simulink model "DirectSequenceSpreadSpectrumCommunicationSystemSimulation"  (R2023a)
settings: Solver=VariableStepAuto  StartTime=0.0  StopTime=10  RelTol=1e-3
InitFcn:
  | fs=1e4;
  | Ts=1/fs;
  | Tb=0.1;
  | Tc=0.0125;
  | frame_size=1000;
libraries: commdigbbndpm3 x4, dspsrcs4 x4, commrandsrc3 x2, commfilt2 x2, commchan3 x1, dspstat3 x1
settings Model: Creator=STUDENT  LastModifiedBy=LENOVO
settings SolverCC: AlgebraicLoopSolver=TrustRegion
settings DebuggingCC: UnconnectedInputMsg=warning  UnconnectedOutputMsg=warning  UnconnectedLineMsg=warning
settings ModelReferenceCC: EnableRefExpFcnMdlSchedulingChecks=on
settings SFSimCC: CustomCodeUndefinedFunction=UseInterfaceOnly

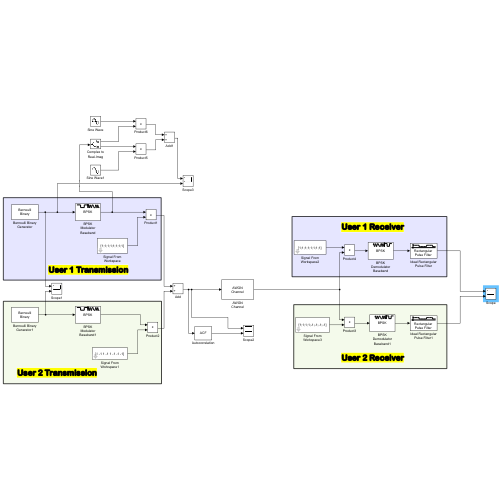
[thumbnail: Simulink's stored preview of the top-level diagram]
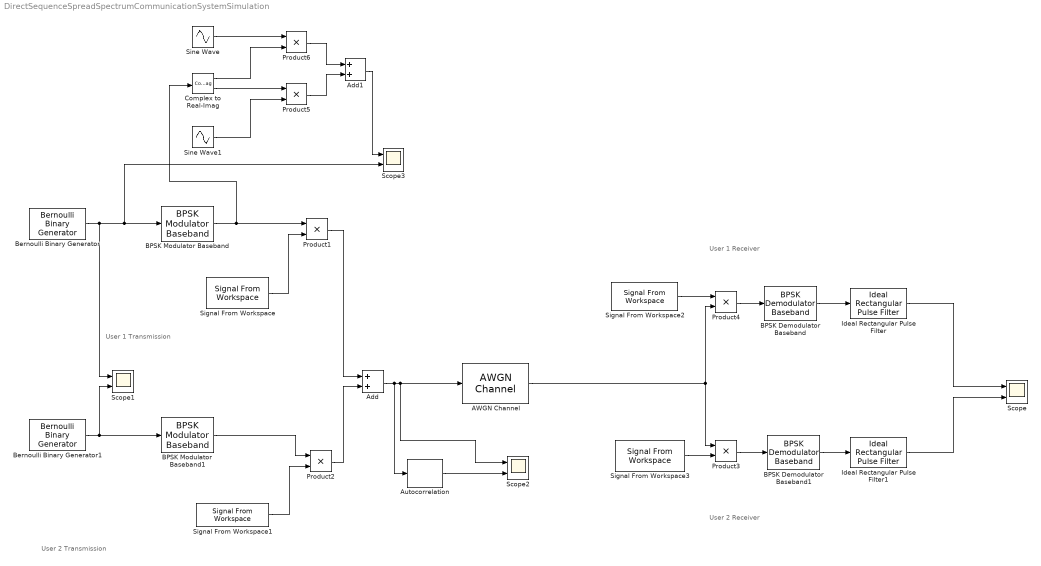
== system DirectSequenceSpreadSpectrumCommunicationSystemSimulation ==
  note: User 1 Transmission
  note: User 2 Transmission
  note: User 1 Receiver
  note: User 2 Receiver
  AWGN Channel : commchan3/AWGN Channel  LegacyMode=on  NoiseMethod="Signal to noise ratio  (SNR)"  noiseMode=Variance from mask  EbNo=10  EsNo=10  SNR=10  BitsPerSymbol=1  SignalPower=1  SamplesPerSymbol=1  SymbolPeriod=1  VarianceSource=Parameter  Variance=10  RandomStream=Global stream  Seed=67  SimulateUsing=Code generation
  Add : Sum
  Add1 : Sum
  Autocorrelation : dspstat3/Autocorrelation  AllPositiveLags=on  maxlag=1  bias=None  domain=Time  roundingMode=Floor  overflowMode=off  outputDataTypeStr=Inherit: Same as accumulator  outputMin=[]  outputMax=[]  outputLastDataTypeStr=Inherit: Same as accumulator
  BPSK Demodulator Baseband : commdigbbndpm3/BPSK Demodulator Baseband  DecType=Hard decision  VarSource=Dialog  Variance=1  Ph=0  outDtype=Inherit via internal rule  derotateFactorWordLen=16  derotateFactorDataTypeStr=Inherit: Same word length as input  derotateFactorLastDataTypeStr=Inherit: Same word length as input
  BPSK Demodulator Baseband1 : commdigbbndpm3/BPSK Demodulator Baseband  DecType=Hard decision  VarSource=Dialog  Variance=1  Ph=0  outDtype=Inherit via internal rule  derotateFactorWordLen=16  derotateFactorDataTypeStr=Inherit: Same word length as input  derotateFactorLastDataTypeStr=Inherit: Same word length as input
  BPSK Modulator Baseband : commdigbbndpm3/BPSK Modulator Baseband  Ph=0  outDtype=double  outWordLen=16  outUDDataType=sfix(16)  outFracLenMode=Best precision  outFracLen=15  outDataTypeStr=double  outLastDataTypeStr=double
  BPSK Modulator Baseband1 : commdigbbndpm3/BPSK Modulator Baseband  Ph=0  outDtype=double  outWordLen=16  outUDDataType=sfix(16)  outFracLenMode=Best precision  outFracLen=15  outDataTypeStr=double  outLastDataTypeStr=double
  Bernoulli Binary Generator : commrandsrc3/Bernoulli Binary Generator  ProbabilityOfZero=0.5  SeedSource=Auto  Seed=0  SampleTime=Tb  SamplesPerFrame=1  OutputDataType=double  SimulateUsing=Interpreted execution
  Bernoulli Binary Generator1 : commrandsrc3/Bernoulli Binary Generator  ProbabilityOfZero=0.5  SeedSource=Auto  Seed=0  SampleTime=Tb  SamplesPerFrame=1  OutputDataType=double  SimulateUsing=Interpreted execution
  Complex to Real-Imag : ComplexToRealImag
  Ideal Rectangular Pulse Filter : commfilt2/Ideal Rectangular Pulse Filter  pulseLen=8  pulseDelay=0  InputProcessing=Columns as channels (frame based)  RateOptions=Enforce single-rate processing  sampMode=Mute  normCheck=off  normMode=Sum of samples  filterGain=1  saveAsFlag=0  roundingMode=Floor  overflowMode=off  firstCoeffDataTypeStr=Inherit: Same word length as input  firstCoeffMin=[]  firstCoeffMax=[]  firstCoeffLastDataTypeStr=Inherit: Same word length as input  outputDataTypeStr=Inherit: Same as accumulator  outputMin=[]  outputMax=[]  outputLastDataTypeStr=Inherit: Same as accumulator
  Ideal Rectangular Pulse Filter1 : commfilt2/Ideal Rectangular Pulse Filter  pulseLen=8  pulseDelay=0  InputProcessing=Columns as channels (frame based)  RateOptions=Enforce single-rate processing  sampMode=Mute  normCheck=off  normMode=Sum of samples  filterGain=1  saveAsFlag=0  roundingMode=Floor  overflowMode=off  firstCoeffDataTypeStr=Inherit: Same word length as input  firstCoeffMin=[]  firstCoeffMax=[]  firstCoeffLastDataTypeStr=Inherit: Same word length as input  outputDataTypeStr=Inherit: Same as accumulator  outputMin=[]  outputMax=[]  outputLastDataTypeStr=Inherit: Same as accumulator
  Product{1..6} (6 alike) : Product
  Scope{,1..3} (4 alike) : Scope  NumInputPorts=2
  Signal From Workspace : dspsrcs4/Signal From Workspace  X=[1;1;1;1;1;1;1;1]  Ts=1  nsamps=1  OutputAfterFinalValue=Setting to zero  ignoreOrWarnInputAndFrameLengths=off  OutputFrames=off
  Signal From Workspace1 : dspsrcs4/Signal From Workspace  X=[1 -1 1 -1 1 -1 -1 -1]  Ts=1  nsamps=1  OutputAfterFinalValue=Setting to zero  ignoreOrWarnInputAndFrameLengths=off  OutputFrames=off
  Signal From Workspace2 : dspsrcs4/Signal From Workspace  X=[1;1;1;1;1;1;1;1]  Ts=1  nsamps=1  OutputAfterFinalValue=Setting to zero  ignoreOrWarnInputAndFrameLengths=off  OutputFrames=off
  Signal From Workspace3 : dspsrcs4/Signal From Workspace  X=[1;1;1;1;-1;-1;-1;-1]  Ts=1  nsamps=1  OutputAfterFinalValue=Setting to zero  ignoreOrWarnInputAndFrameLengths=off  OutputFrames=off
  Sine Wave : Sin  Frequency=8*pi  SampleTime=0.001
  Sine Wave1 : Sin  Frequency=8*pi  Phase=pi/2  SampleTime=0.001
  wires:
  Bernoulli Binary Generator1/1 -> BPSK Modulator Baseband1/1, Scope1/2
  Product3/1 -> BPSK Demodulator Baseband1/1
  BPSK Demodulator Baseband1/1 -> Ideal Rectangular Pulse Filter1/1
  BPSK Demodulator Baseband/1 -> Ideal Rectangular Pulse Filter/1
  BPSK Modulator Baseband/1 -> Complex to Real-Imag/1, Product1/1
  Product1/1 -> Add/1
  Signal From Workspace1/1 -> Product2/2
  BPSK Modulator Baseband1/1 -> Product2/1
  Product2/1 -> Add/2
  Signal From Workspace2/1 -> Product4/1
  Signal From Workspace3/1 -> Product3/2
  AWGN Channel/1 -> Product4/2, Product3/1
  Product4/1 -> BPSK Demodulator Baseband/1
  Ideal Rectangular Pulse Filter/1 -> Scope/1
  Add/1 -> Scope2/1, AWGN Channel/1, Autocorrelation/1
  Sine Wave/1 -> Product6/1
  Complex to Real-Imag/1 -> Product6/2
  Complex to Real-Imag/2 -> Product5/1
  Sine Wave1/1 -> Product5/2
  Product6/1 -> Add1/1
  Product5/1 -> Add1/2
  Add1/1 -> Scope3/1
  Bernoulli Binary Generator/1 -> BPSK Modulator Baseband/1, Scope3/2, Scope1/1
  Ideal Rectangular Pulse Filter1/1 -> Scope/2
  Autocorrelation/1 -> Scope2/2
  Signal From Workspace/1 -> Product1/2
